simulink model "Interceptor6DOF"  (R2026a)
settings: Solver=ode45  StopTime=20  MaxStep=0.01  RelTol=1e-6
settings Model: Creator=AYUSH  LastModifiedBy=AYUSH

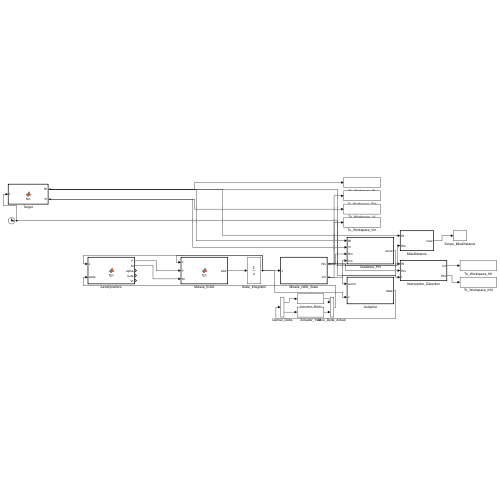
[thumbnail: Simulink's stored preview of the top-level diagram]
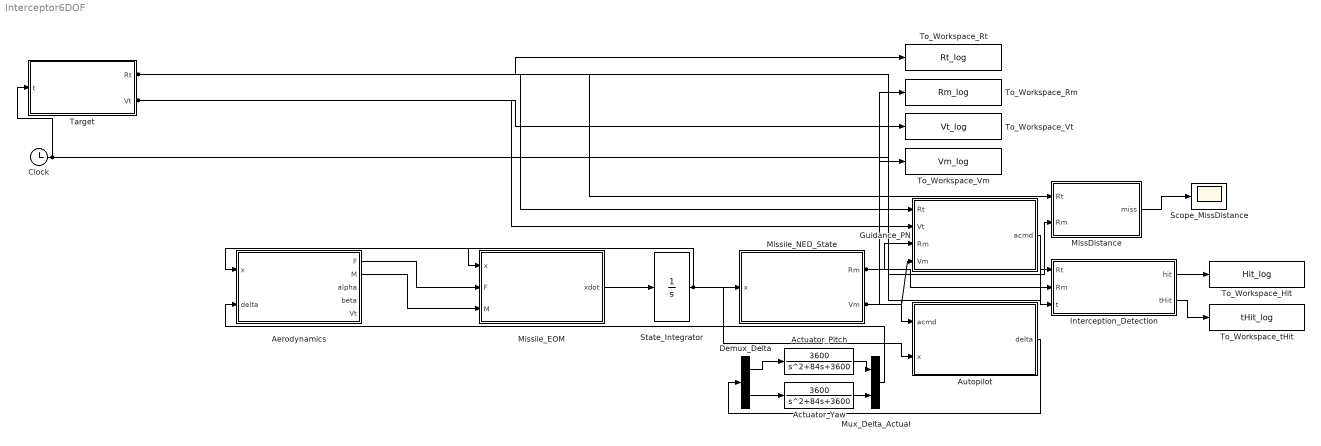
== system Interceptor6DOF ==
  Actuator_Pitch : TransferFcn  Numerator=[3600]  Denominator=[1 84 3600]
  Actuator_Yaw : TransferFcn  Numerator=[3600]  Denominator=[1 84 3600]
  Aerodynamics : MATLAB Function  TreatAsAtomicUnit=on
  Autopilot : MATLAB Function  TreatAsAtomicUnit=on
  Clock : Clock
  Demux_Delta : Demux  Outputs=2
  Guidance_PN : MATLAB Function  TreatAsAtomicUnit=on
  Interception_Detection : MATLAB Function  TreatAsAtomicUnit=on
  MissDistance : MATLAB Function  TreatAsAtomicUnit=on
  Missile_EOM : MATLAB Function  TreatAsAtomicUnit=on
  Missile_NED_State : MATLAB Function  TreatAsAtomicUnit=on
  Mux_Delta_Actual : Mux  Inputs=2
  Scope_MissDistance : Scope
  State_Integrator : Integrator  InitialCondition=[350;0;0;0;0;0; 0;15*pi/180;0; 0;0;0]
  Target : MATLAB Function  TreatAsAtomicUnit=on
  To_Workspace_Hit : ToWorkspace  VariableName=Hit_log  SaveFormat=Structure With Time  SampleTime=-1
  To_Workspace_Rm : ToWorkspace  VariableName=Rm_log  SaveFormat=Structure With Time  SampleTime=-1
  To_Workspace_Rt : ToWorkspace  VariableName=Rt_log  SaveFormat=Structure With Time  SampleTime=-1
  To_Workspace_Vm : ToWorkspace  VariableName=Vm_log  SaveFormat=Structure With Time  SampleTime=-1
  To_Workspace_Vt : ToWorkspace  VariableName=Vt_log  SaveFormat=Structure With Time  SampleTime=-1
  To_Workspace_tHit : ToWorkspace  VariableName=tHit_log  SaveFormat=Structure With Time  SampleTime=-1
  wires:
  Clock/1 -> Target/1(t), Interception_Detection/3(t)
  Target/1(Rt) -> Guidance_PN/1(Rt), MissDistance/1(Rt), To_Workspace_Rt/1, Interception_Detection/1(Rt)
  Target/2(Vt) -> Guidance_PN/2(Vt), To_Workspace_Vt/1
  State_Integrator/1 -> Missile_NED_State/1(x), Autopilot/2(x), Aerodynamics/1(x), Missile_EOM/1(x)
  Missile_NED_State/1(Rm) -> Guidance_PN/3(Rm), MissDistance/2(Rm), To_Workspace_Rm/1, Interception_Detection/2(Rm)
  Missile_NED_State/2(Vm) -> Guidance_PN/4(Vm), To_Workspace_Vm/1
  Guidance_PN/1(acmd) -> Autopilot/1(acmd)
  Autopilot/1(delta) -> Demux_Delta/1
  Demux_Delta/1 -> Actuator_Pitch/1
  Demux_Delta/2 -> Actuator_Yaw/1
  Actuator_Pitch/1 -> Mux_Delta_Actual/1
  Actuator_Yaw/1 -> Mux_Delta_Actual/2
  Mux_Delta_Actual/1 -> Aerodynamics/2(delta)
  Aerodynamics/1(F) -> Missile_EOM/2(F)
  Aerodynamics/2(M) -> Missile_EOM/3(M)
  Missile_EOM/1(xdot) -> State_Integrator/1
  MissDistance/1(miss) -> Scope_MissDistance/1
  Interception_Detection/1(hit) -> To_Workspace_Hit/1
  Interception_Detection/2(tHit) -> To_Workspace_tHit/1

== matlab function Interceptor6DOF/Missile_EOM ==
  data: x input; xdot output; F input; M input
function xdot = fcn(x, F, M)
%#codegen
% Generic small-interceptor mass properties (tune with real data)
m    = 120;      % kg
Ixx  = 8;         % kg*m^2 (roll)
Iyy  = 55;        % kg*m^2 (pitch)
Izz  = 55;        % kg*m^2 (yaw)
g0   = 9.81;

u=x(1); v=x(2); w=x(3);
p=x(4); q=x(5); r=x(6);
phi=x(7); theta=x(8); psi=x(9);

Fx=F(1); Fy=F(2); Fz=F(3);
Mx=M(1); My=M(2); Mz=M(3);

% gravity resolved into body axes
gx = -g0*sin(theta);
gy =  g0*cos(theta)*sin(phi);
gz =  g0*cos(theta)*cos(phi);

udot = Fx/m + gx - q*w + r*v;
vdot = Fy/m + gy - r*u + p*w;
wdot = Fz/m + gz - p*v + q*u;

pdot = ((Iyy-Izz)/Ixx)*q*r + Mx/Ixx;
qdot = ((Izz-Ixx)/Iyy)*p*r + My/Iyy;
rdot = ((Ixx-Iyy)/Izz)*p*q + Mz/Izz;

phidot   = p + tan(theta)*(q*sin(phi)+r*cos(phi));
thetadot = q*cos(phi) - r*sin(phi);
psidot   = (q*sin(phi)+r*cos(phi))/cos(theta);

cphi=cos(phi); sphi=sin(phi);
cth=cos(theta); sth=sin(theta);
cpsi=cos(psi); spsi=sin(psi);
DCM = [cth*cpsi, sphi*sth*cpsi-cphi*spsi, cphi*sth*cpsi+sphi*spsi;
       cth*spsi, sphi*sth*spsi+cphi*cpsi, cphi*sth*spsi-sphi*cpsi;
       -sth,      sphi*cth,                cphi*cth];
posdot = DCM*[u;v;w];

xdot = [udot;vdot;wdot;pdot;qdot;rdot;phidot;thetadot;psidot;posdot];
end

== matlab function Interceptor6DOF/Target ==
  data: t input; Rt output; Vt output
function [Rt, Vt] = fcn(t)
%#codegen
% Non-maneuvering target starting 6000 m north, 3000 m altitude,
% closing at 250 m/s toward the missile launch point.
R0 = [5000; 500; -3000];   % NED: [North; East; Down] (Down negative = up)
V0 = [-250; 10; 20];         % constant velocity, m/s
Rt = R0 + V0*t;
Vt = V0;
end

== matlab function Interceptor6DOF/Missile_NED_State ==
  data: x input; Rm output; Vm output
function [Rm, Vm] = fcn(x)
%#codegen
u=x(1); v=x(2); w=x(3);
phi=x(7); theta=x(8); psi=x(9);
cphi=cos(phi); sphi=sin(phi);
cth=cos(theta); sth=sin(theta);
cpsi=cos(psi); spsi=sin(psi);
DCM = [cth*cpsi, sphi*sth*cpsi-cphi*spsi, cphi*sth*cpsi+sphi*spsi;
       cth*spsi, sphi*sth*spsi+cphi*cpsi, cphi*sth*spsi-sphi*cpsi;
       -sth,      sphi*cth,                cphi*cth];
Rm = x(10:12);
Vm = DCM*[u;v;w];
end

== matlab function Interceptor6DOF/Guidance_PN ==
  data: Rt input; acmd output; Vt input; Rm input; Vm input
function acmd = fcn(Rt, Vt, Rm, Vm)
%#codegen
N = 4;                            % navigation constant
Rrel = Rt - Rm;
Vrel = Vt - Vm;
r2 = dot(Rrel,Rrel);
if r2 < 1
    r2 = 1;                        % avoid singularity near intercept
end
omega = cross(Rrel, Vrel) / r2;   % LOS rotation rate vector
Vc = -dot(Rrel,Vrel)/sqrt(r2);    % closing velocity

% ---> GRAVITY COMPENSATION ADDED HERE <--- 
acmd = N * Vc * cross(omega, Rrel/sqrt(r2)) + [0; 0; -9.81];
end

== matlab function Interceptor6DOF/Autopilot ==
  data: acmd input; delta output; x input
function delta = fcn(acmd, x)
%#codegen
% Calculate Dynamic Pressure (qbar) for gain scheduling
u=x(1); v=x(2); w=x(3);
Vt = sqrt(u^2+v^2+w^2);
if Vt < 1, Vt = 1; end
rho = 1.225 * exp(x(12)/8500);    % Air density at current altitude (-Z)
qbar = 0.5 * rho * Vt^2;

phi=x(7); theta=x(8); psi=x(9);
cphi=cos(phi); sphi=sin(phi);
cth=cos(theta); sth=sin(theta);
cpsi=cos(psi); spsi=sin(psi);
DCM = [cth*cpsi, sphi*sth*cpsi-cphi*spsi, cphi*sth*cpsi+sphi*spsi;
       cth*spsi, sphi*sth*spsi+cphi*cpsi, cphi*sth*spsi-sphi*cpsi;
       -sth,      sphi*cth,                cphi*cth];
a_body = DCM.'*acmd;              % NED->body

% Auto-tune Kp using Mass / (22 * Sref) so it tracks perfectly 1-to-1
Kp = 174 / qbar;

delta_pitch = Kp * a_body(3);
delta_yaw   = Kp * a_body(2);

maxDef = 20*pi/180;
delta_pitch = max(min(delta_pitch, maxDef), -maxDef);
delta_yaw   = max(min(delta_yaw,   maxDef), -maxDef);

delta = [delta_pitch; delta_yaw];
end

== matlab function Interceptor6DOF/Aerodynamics ==
  data: x input; F output; delta input; M output; alpha output; beta output; Vt output
function [F, M, alpha, beta, Vt] = fcn(x, delta)
%#codegen
% Generic linear missile aero model + boost/sustain thrust.
u=x(1); v=x(2); w=x(3); q=x(5); r=x(6);
zpos = x(12);

Vt = sqrt(u^2+v^2+w^2);
if Vt < 1
    Vt = 1;
end
alpha = atan2(w,u);
beta  = asin(max(min(v/Vt,1),-1));

% simple exponential atmosphere
alt = -zpos;
rho0 = 1.225; H = 8500;
rho = rho0*exp(-alt/H);
qbar = 0.5*rho*Vt^2;

Sref = 0.0314;   % m^2, reference area (~200mm diameter body)
d    = 0.2;      % m, reference length

% aero coefficients (generic, linear)
CNalpha = 12; CNdelta = 8;
CYbeta  = -12; CYdelta = -8;
Cmalpha = -4;  Cmdelta = -10; Cmq = -200;
Cnbeta  = 4;   Cndelta = 10;  Cnr = -200;
CA0 = 0.3;      % axial drag coefficient

delta_p = delta(1); delta_y = delta(2);

CN = CNalpha*alpha + CNdelta*delta_p;
CY = CYbeta*beta   + CYdelta*delta_y;
CA = CA0;

Cm = Cmalpha*alpha + Cmdelta*delta_p + Cmq*q*d/(2*Vt);
Cn = Cnbeta*beta   + Cndelta*delta_y + Cnr*r*d/(2*Vt);
Cl = 0;   % no roll control modeled

% simple boost-sustain thrust profile (illustrative only)
thrust = 400;   % N, constant sustain thrust along body x-axis

Fx = -qbar*Sref*CA + thrust;
Fy =  qbar*Sref*CY;
Fz = -qbar*Sref*CN;

Mx = qbar*Sref*d*Cl;
My = qbar*Sref*d*Cm;
Mz = qbar*Sref*d*Cn;

F = [Fx;Fy;Fz];
M = [Mx;My;Mz];
end

== matlab function Interceptor6DOF/MissDistance ==
  data: Rt input; miss output; Rm input
function miss=fcn(Rt,Rm)
%#codegen
miss=norm(Rt-Rm);
end

== matlab function Interceptor6DOF/Interception_Detection ==
  data: Rt input; hit output; Rm input; t input; tHit output
function [hit,tHit]=fcn(Rt,Rm,t)
%#codegen
if norm(Rt-Rm)<=10
 hit=1; tHit=t;
else
 hit=0; tHit=-1;
end
end
